simulink model "relop_multi_test"  (Simulink 9.0)
settings: Solver=FixedStepAuto  StartTime=0.0  StopTime=10.0  FixedStep=1.000000  RelTol=1e-3  EnableMultiTasking=on
settings Model: SuppressorTable=22 serialization::archive 11 0 6 0 0 0 0 0  Creator=arnaud  LastModifiedBy=hbourbou
settings DataIOCC: LimitDataPoints=on  SaveFormat=Structure  SignalLoggingSaveFormat=ModelDataLogs
settings OptimizationCC: ExpressionDepthLimit=2147483647
settings DebuggingCC: SolverPrmCheckMsg=warning  FcnCallInpInsideContextMsg=warning  StateNameClashWarn=warning  StrictBusMsg=Warning
settings GRTTargetCC: CombineOutputUpdateFcns=off  GRTInterface=on

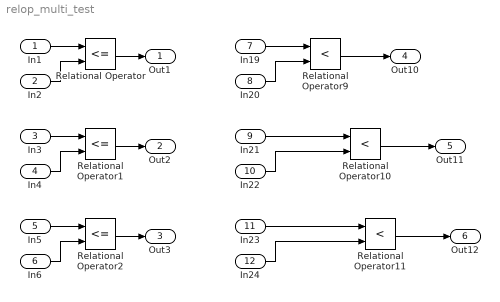
== system relop_multi_test ==
  In1 : Inport  OutDataTypeStr=double  PortDimensions=3
  In2 : Inport  Port=2  OutDataTypeStr=double  PortDimensions=3
  In3 : Inport  Port=3  OutDataTypeStr=int8  PortDimensions=3
  In4 : Inport  Port=4  OutDataTypeStr=int8  PortDimensions=1
  In5 : Inport  Port=5  OutDataTypeStr=boolean  PortDimensions=1
  In6 : Inport  Port=6  OutDataTypeStr=boolean  PortDimensions=3
  In19 : Inport  Port=7  OutDataTypeStr=double  PortDimensions=[2 3]
  In20 : Inport  Port=8  OutDataTypeStr=double  PortDimensions=1
  In21 : Inport  Port=9  OutDataTypeStr=int8  PortDimensions=1
  In22 : Inport  Port=10  OutDataTypeStr=int8  PortDimensions=[2 3]
  In23 : Inport  Port=11  OutDataTypeStr=boolean  PortDimensions=[2 3]
  In24 : Inport  Port=12  OutDataTypeStr=boolean  PortDimensions=[2 3]
  Relational Operator : RelationalOperator  Operator=<=  OutDataTypeStr=boolean  RndMeth=Nearest
  Relational Operator1 : RelationalOperator  Operator=<=  OutDataTypeStr=boolean  RndMeth=Nearest
  Relational Operator10 : RelationalOperator  Operator=<  OutDataTypeStr=boolean  RndMeth=Nearest
  Relational Operator11 : RelationalOperator  Operator=<  OutDataTypeStr=boolean  RndMeth=Nearest
  Relational Operator2 : RelationalOperator  Operator=<=  OutDataTypeStr=boolean  RndMeth=Nearest
  Relational Operator9 : RelationalOperator  Operator=<  OutDataTypeStr=boolean  RndMeth=Nearest
  Out1 : Outport
  Out2 : Outport  Port=2
  Out3 : Outport  Port=3
  Out10 : Outport  Port=4
  Out11 : Outport  Port=5
  Out12 : Outport  Port=6
  wires:
  In1/1 -> Relational Operator/1
  Relational Operator/1 -> Out1/1
  In2/1 -> Relational Operator/2
  In3/1 -> Relational Operator1/1
  Relational Operator1/1 -> Out2/1
  In4/1 -> Relational Operator1/2
  In5/1 -> Relational Operator2/1
  Relational Operator2/1 -> Out3/1
  In6/1 -> Relational Operator2/2
  In19/1 -> Relational Operator9/1
  Relational Operator9/1 -> Out10/1
  In20/1 -> Relational Operator9/2
  In21/1 -> Relational Operator10/1
  Relational Operator10/1 -> Out11/1
  In22/1 -> Relational Operator10/2
  In23/1 -> Relational Operator11/1
  Relational Operator11/1 -> Out12/1
  In24/1 -> Relational Operator11/2
